simulink model "Bebop2_sim_only_vis"  (R2018a)
settings: Solver=VariableStepAuto  StartTime=0.0  StopTime=20  FixedStep=.05  MaxStep=1  MinStep=0.1  RelTol=50  AbsTol=50
values from neighbouring files (symbols this model uses):
  flightplan = [dist,0,height,deg2rad(090) ... (first row only)    [compare_cubic_spline_1.m]    (also in initialize_race_realtime.m; initialize_race_realtime_backup_cubic.m; plot_sim.m = [ 4.348, -0.278, height, deg2rad(  0); test_b_spline.m)
  FOV = 1.05    [initialize_race_realtime.m]    (also in initialize_race_realtime_backup_cubic.m)
  g = 9.81    [initialize_race_no_realtime.m]    (also in initialize_race_realtime.m; initialize_race_realtime_backup_cubic.m; moving_average_rls_own.m = P(i-1)*meas*(lambda+meas*P(i-1)*meas)^-1)
  gate_size = 1.4    [initialize_race_realtime.m]    (also in initialize_race_realtime_backup_cubic.m)
  gates = sim_gates(:,:,1)    [eval_sim.m]    (also in initialize_race_realtime.m = [dist,0,height,deg2rad(110); initialize_race_realtime_backup_cubic.m = [dist,0,height,deg2rad(110); plot_sim.m)
  init_std_dev = [1.0*ones(1,3),deg2rad(30)]    [initialize_race_realtime.m]    (also in initialize_race_realtime_backup_cubic.m)
  Initial_ori = [0 0 pi/4]    [initialize_race_no_realtime.m]    (also in initialize_race_realtime.m; initialize_race_realtime_backup_cubic.m)
  Initial_pos = [0 0 1]    [Bebop_sim_init.m]    (also in initialize_race_no_realtime.m = [0 -3 2]; initialize_race_realtime.m = [0 -3 2]; initialize_race_realtime_backup_cubic.m = [0 -3 2])
  Initial_vel_e = max_vel*[1,0,0]    [initialize_race_realtime.m]    (also in initialize_race_realtime_backup_cubic.m)
  max_rot_Z = (90)*pi/180    (= 1.57079632679)    [Bebop_sim_init.m]    (also in initialize_race_no_realtime.m = 1.0471975512; initialize_race_realtime.m; initialize_race_realtime_backup_cubic.m; run_batch1.m = list_agility(idx_agility)*max_rot_Z)
  max_theta_X = (40)*pi/180    (= 0.698131700798)    [Bebop_sim_init.m]    (also in initialize_race_no_realtime.m = 0.13962634016; initialize_race_realtime.m = 1.308996939; initialize_race_realtime_backup_cubic.m = 1.308996939; run_batch1.m = list_agility(idx_agility)*max_theta_X)
  max_theta_Y = (40)*pi/180    (= 0.698131700798)    [Bebop_sim_init.m]    (also in initialize_race_no_realtime.m = 0.13962634016; initialize_race_realtime.m = 1.308996939; initialize_race_realtime_backup_cubic.m = 1.308996939; run_batch1.m = list_agility(idx_agility)*max_theta_Y)
  max_v_Z = .5    (= 0.5)    [Bebop_sim_init.m]    (also in initialize_race_no_realtime.m = 1; initialize_race_realtime.m = 3; initialize_race_realtime_backup_cubic.m = 3; run_batch1.m = list_agility(idx_agility)*max_v_Z)
  max_vel = 1.5    [initialize_race_realtime.m]    (also in initialize_race_realtime_backup_cubic.m; run_batch1.m = list_speed(idx_speed); run_batch2.m = list_speed(idx_speed); run_batch3.m = list_speed(idx_speed))
undefined symbols (not defined in the file or in its folder): fspecial, gray, Rec, SDTV
libraries: sharedtransform x9, simulink x4, visiontextngfix x4, visiontransforms x3, vrlib x2, visionanalysis x2, visionconversions x2, aerolibutil x1, visionstatistics x1, visionsinks x1
(part 1 of 2)
settings Model: EnablePacing=on  Creator=vinni  LastModifiedBy=vinni
settings HardwareCC: ProdBitPerLong=64  ProdHWDeviceType=Intel->x86-64 (Linux 64)

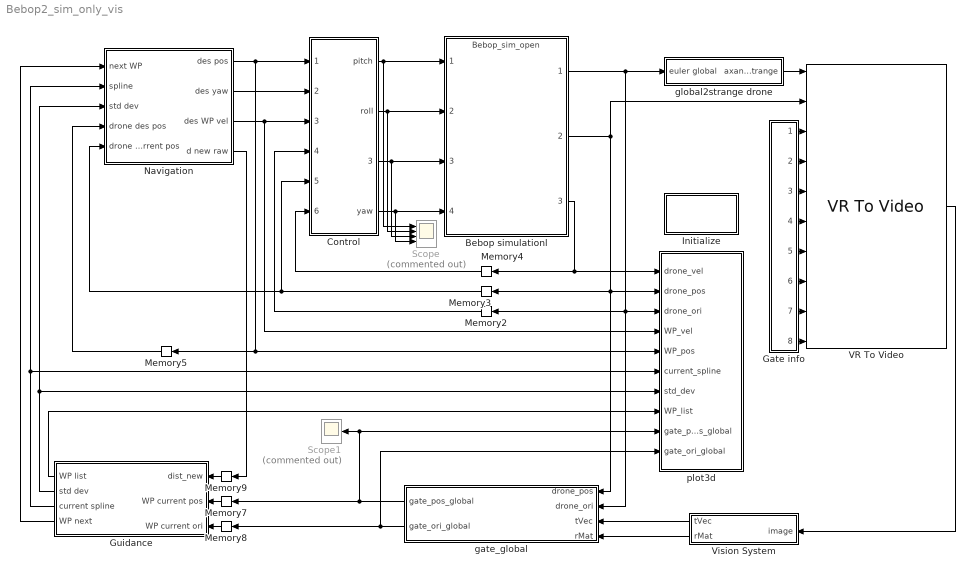
== system Bebop2_sim_only_vis ==
  Bebop simulationl : ModelReference  ModelNameDialog=Bebop_sim_open.slx  SimulationMode=Normal  ModelReferenceVersion=1.35
  Control : Subsystem
  Gate info : Subsystem
  Guidance : Subsystem
  Initialize : Subsystem  TreatAsAtomicUnit=on
  Memory2 : Memory  InitialCondition=Initial_ori
  Memory3 : Memory  InitialCondition=Initial_pos
  Memory4 : Memory  InitialCondition=Initial_vel_e
  Memory5 : Memory
  Memory7 : Memory
  Memory8 : Memory  InitialCondition=zeros(1,3)
  Memory9 : Memory
  Navigation : Subsystem
  Scope : Scope  Commented=on  NumInputPorts=4
  Scope1 : Scope  Commented=on
  VR To Video : vrlib/VR To Video  InstantiateOnLoad=on  SampleTime=0.1000001  ViewEnable=on  RemoteChange=off  RemoteView=off  FieldsWritten=drone.orientation.4.1.1.double#drone.position.3.1.1.double#G1.rotation.4.1.1.double#G1.translation.3.1.1.double#G2.rotation.4.1.1.double#G2.translation.3.1.1.double#G3.rotation.4.1.1.double#G3.translation.3.1.1.double#G4.rotation.4.1.1.double#G4.translation.3.1.1.double  WorldFileName=race_course.wrl  AutoView=off  VideoDimensions=1.5*[200 320]  AllowVariableSize=off  FigureProperties="{'Position', 'Name', 'Viewpoint', 'CameraBound', 'CameraDirection', 'CameraPosition', 'CameraUpVector', 'ZoomFactor', 'Antialiasing', 'Headlight', 'Lighting', 'NavPanel', 'Sound', 'StatusBar', 'Stereo3D', 'Stereo3DCameraOffset', 'Stereo3DHIT', 'ToolBar', 'Textures', 'Transparency', 'Triad', 'Wireframe', 'NavZones', 'NavMode', 'NavSpeed', 'CaptureFileFormat', 'CaptureFileName', 'Record2DCompressMethod', 'Record2DCompressQuality', 'Record2D', 'Record2DFileName', 'Record2DFPS'; [3.0000000000000000e+01   6.0000000000000000e+01   4.8000000000000000e+02   3.0000000000000000e+02], '', '_untitled_1', 'on', [0.0000000000000000e+00   0.0000000000000000e+00  -1.0000000000000000e+00], [0.0000000000000000e+00   0.0000000000000000e+00   0.0000000000000000e+00], [0.0000000000000000e+00   1.0000000000000000e+00   0.0000000000000000e+00], [1.0000000000000000e+00], 'on', 'on', 'on', 'none', 'on', 'off', 'off', [1.0000000149011612e-01], [0.0000000000000000e+00], 'off', 'on', 'on', 'none', 'off', 'off', 'fly', 'normal', 'tif', '%f_anim_%n.tif', 'auto', [7.5000000000000000e+01], 'off', '***video***', 'auto'}"
      settings: SourceProductName=Simulink 3D Animation  SourceProductBaseCode=VR
  Vision System : Subsystem
  gate_global : MATLAB Function  TreatAsAtomicUnit=on
  global2strange drone : Subsystem
  plot3d : MATLAB Function  TreatAsAtomicUnit=on
  wires:
  Bebop simulationl/3 -> plot3d/1(drone_vel), Memory4/1
  Bebop simulationl/2 -> VR To Video/2, Memory3/1, gate_global/1(drone_pos), plot3d/2(drone_pos)
  Bebop simulationl/1 -> global2strange drone/1(euler global), Memory2/1, gate_global/2(drone_ori), plot3d/3(drone_ori)
  gate_global/1(gate_pos_global) -> plot3d/9(gate_pos_global), Scope1/1, Memory7/1
  gate_global/2(gate_ori_global) -> plot3d/10(gate_ori_global), Memory8/1
  VR To Video/1 -> Vision System/1(image)
  Vision System/1(tVec) -> gate_global/3(tVec)
  Vision System/2(rMat) -> gate_global/4(rMat)
  Control/4(yaw) -> Bebop simulationl/4, Scope/4
  Control/3(throttle) -> Bebop simulationl/3, Scope/3
  Control/2(roll) -> Bebop simulationl/2, Scope/2
  Control/1(pitch) -> Bebop simulationl/1, Scope/1
  Memory4/1 -> Control/6(Drone vel)
  Memory2/1 -> Control/4(Drone ori)
  Guidance/3(current spline) -> Navigation/2(spline), plot3d/6(current_spline)
  Memory7/1 -> Guidance/2(WP current pos)
  Memory8/1 -> Guidance/3(WP current ori)
  Memory9/1 -> Guidance/1(dist_new)
  Guidance/1(WP list) -> plot3d/8(WP_list)
  global2strange drone/1(axang strange) -> VR To Video/1
  Gate info/2(P1) -> VR To Video/4
  Gate info/4(P2) -> VR To Video/6
  Gate info/6(P3) -> VR To Video/8
  Gate info/8(P4) -> VR To Video/10
  Gate info/1(O1) -> VR To Video/3
  Gate info/3(O2) -> VR To Video/5
  Gate info/5(O3) -> VR To Video/7
  Gate info/7(O4) -> VR To Video/9
  Memory3/1 -> Control/5(Drone pos), Navigation/5(drone current pos)
  Guidance/2(std dev) -> plot3d/7(std_dev), Navigation/3(std dev)
  Navigation/1(des pos) -> Control/1(WP pos), plot3d/5(WP_pos), Memory5/1
  Navigation/3(des WP vel) -> Control/3(WP vel), plot3d/4(WP_vel)
  Memory5/1 -> Navigation/4(drone des pos)
  Guidance/4(WP next) -> Navigation/1(next WP)
  Navigation/2(des yaw) -> Control/2(des yaw)
  Navigation/4(d new raw) -> Memory9/1

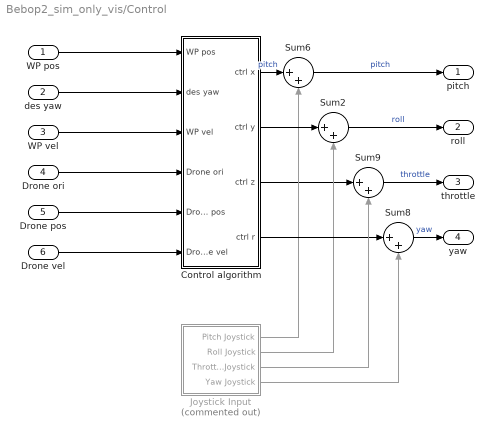
== system Bebop2_sim_only_vis/Control ==
  WP pos : Inport
  des yaw : Inport  Port=2
  WP vel : Inport  Port=3
  Drone ori : Inport  Port=4
  Drone pos : Inport  Port=5
  Drone vel : Inport  Port=6
  Control algorithm : Subsystem
  Joystick Input : Subsystem  Commented=on
  Sum{2,6,8..9} (4 alike) : Sum  Inputs=|++
  pitch : Outport
  roll : Outport  Port=2
  throttle : Outport  Port=3
  yaw : Outport  Port=4
  wires:
  Drone ori/1 -> Control algorithm/4(Drone ori)
  Control algorithm/3(ctrl z) -> Sum9/1
  Joystick Input/2(Roll Joystick) -> Sum2/2
  Joystick Input/4(Yaw Joystick) -> Sum8/2
  Drone pos/1 -> Control algorithm/5(Drone pos)
  Joystick Input/1(Pitch Joystick) -> Sum6/2
  des yaw/1 -> Control algorithm/2(des yaw)
  Sum8/1 -> yaw/1  "yaw"
  Sum6/1 -> pitch/1  "pitch"
  Control algorithm/2(ctrl y) -> Sum2/1
  WP pos/1 -> Control algorithm/1(WP pos)
  Control algorithm/4(ctrl r) -> Sum8/1
  Sum2/1 -> roll/1  "roll"
  WP vel/1 -> Control algorithm/3(WP vel)
  Control algorithm/1(ctrl x) -> Sum6/1  "pitch"
  Drone vel/1 -> Control algorithm/6(Drone vel)
  Sum9/1 -> throttle/1  "throttle"
  Joystick Input/3(Throttle Joystick) -> Sum9/2

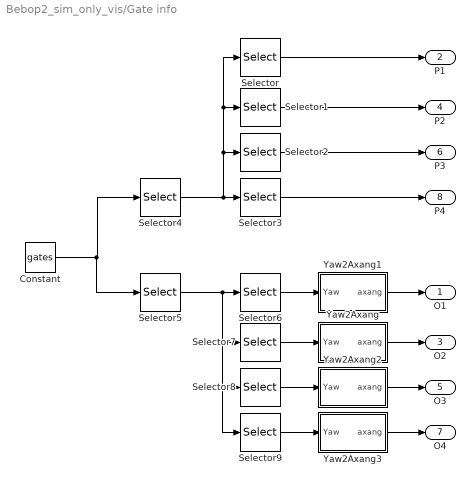
== system Bebop2_sim_only_vis/Gate info ==
  Constant : Constant  Value=gates
  Selector : Selector  NumberOfDimensions=2  InputPortWidth=3  IndexOptions=Index vector (dialog),Select all  Indices=1,1  OutputSizes=1,1
  Selector1 : Selector  NumberOfDimensions=2  InputPortWidth=3  IndexOptions=Index vector (dialog),Select all  Indices=2,1  OutputSizes=1,1
  Selector2 : Selector  NumberOfDimensions=2  InputPortWidth=3  IndexOptions=Index vector (dialog),Select all  Indices=3,1  OutputSizes=1,1
  Selector3 : Selector  NumberOfDimensions=2  InputPortWidth=3  IndexOptions=Index vector (dialog),Select all  Indices=4,1  OutputSizes=1,1
  Selector4 : Selector  NumberOfDimensions=2  InputPortWidth=3  IndexOptions=Select all,Index vector (dialog)  Indices=4,[1 2 3]  OutputSizes=1,1
  Selector5 : Selector  NumberOfDimensions=2  InputPortWidth=3  IndexOptions=Select all,Index vector (dialog)  Indices=4,4  OutputSizes=1,1
  Selector6 : Selector  NumberOfDimensions=2  InputPortWidth=3  IndexOptions=Index vector (dialog),Select all  Indices=1,1  OutputSizes=1,1
  Selector7 : Selector  NumberOfDimensions=2  InputPortWidth=3  IndexOptions=Index vector (dialog),Select all  Indices=2,1  OutputSizes=1,1
  Selector8 : Selector  NumberOfDimensions=2  InputPortWidth=3  IndexOptions=Index vector (dialog),Select all  Indices=3,1  OutputSizes=1,1
  Selector9 : Selector  NumberOfDimensions=2  InputPortWidth=3  IndexOptions=Index vector (dialog),Select all  Indices=4,1  OutputSizes=1,1
  Yaw2Axang : Subsystem
  Yaw2Axang1 : Subsystem
  Yaw2Axang2 : Subsystem
  Yaw2Axang3 : Subsystem
  O1 : Outport
  P1 : Outport  Port=2
  O2 : Outport  Port=3
  P2 : Outport  Port=4
  O3 : Outport  Port=5
  P3 : Outport  Port=6
  O4 : Outport  Port=7
  P4 : Outport  Port=8
  wires:
  Selector/1 -> P1/1
  Selector3/1 -> P4/1
  Selector2/1 -> P3/1
  Selector4/1 -> Selector1/1, Selector/1, Selector2/1, Selector3/1
  Selector1/1 -> P2/1
  Constant/1 -> Selector5/1, Selector4/1
  Selector5/1 -> Selector9/1, Selector8/1, Selector7/1, Selector6/1
  Selector6/1 -> Yaw2Axang1/1(Yaw)
  Selector7/1 -> Yaw2Axang/1(Yaw)
  Selector8/1 -> Yaw2Axang2/1(Yaw)
  Selector9/1 -> Yaw2Axang3/1(Yaw)
  Yaw2Axang1/1(axang) -> O1/1
  Yaw2Axang/1(axang) -> O2/1
  Yaw2Axang2/1(axang) -> O3/1
  Yaw2Axang3/1(axang) -> O4/1

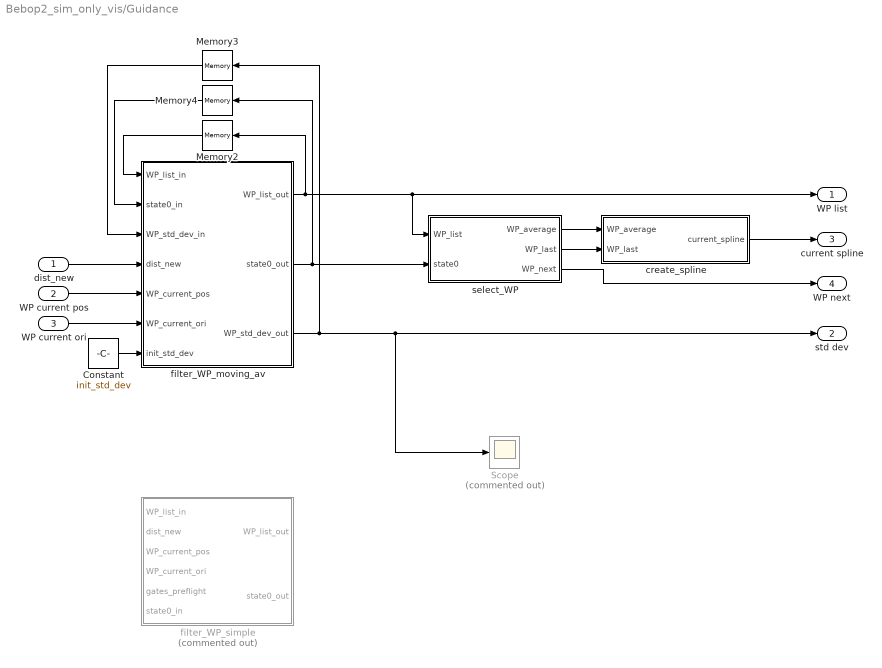
== system Bebop2_sim_only_vis/Guidance ==
  dist_new : Inport
  WP current pos : Inport  Port=2
  WP current ori : Inport  Port=3
  Constant : Constant  Value=init_std_dev
  Memory2 : Memory  InitialCondition=flightplan
  Memory3 : Memory  InitialCondition=init_std_dev
  Memory4 : Memory
  Scope : Scope  Commented=on
  create_spline : MATLAB Function  TreatAsAtomicUnit=on
  filter_WP_moving_av : MATLAB Function  TreatAsAtomicUnit=on
  filter_WP_simple : MATLAB Function  Commented=on  TreatAsAtomicUnit=on
  select_WP : MATLAB Function  TreatAsAtomicUnit=on
  WP list : Outport
  std dev : Outport  Port=2
  current spline : Outport  Port=3
  WP next : Outport  Port=4
  wires:
  WP current ori/1 -> filter_WP_moving_av/6(WP_current_ori)
  create_spline/1(current_spline) -> current spline/1
  select_WP/2(WP_last) -> create_spline/2(WP_last)
  WP current pos/1 -> filter_WP_moving_av/5(WP_current_pos)
  dist_new/1 -> filter_WP_moving_av/4(dist_new)
  select_WP/1(WP_average) -> create_spline/1(WP_average)
  filter_WP_moving_av/1(WP_list_out) -> Memory2/1, WP list/1, select_WP/1(WP_list)
  Memory2/1 -> filter_WP_moving_av/1(WP_list_in)
  filter_WP_moving_av/2(state0_out) -> select_WP/2(state0), Memory4/1
  Memory4/1 -> filter_WP_moving_av/2(state0_in)
  filter_WP_moving_av/3(WP_std_dev_out) -> Scope/1, std dev/1, Memory3/1
  Memory3/1 -> filter_WP_moving_av/3(WP_std_dev_in)
  Constant/1 -> filter_WP_moving_av/7(init_std_dev)
  select_WP/3(WP_next) -> WP next/1

== system Bebop2_sim_only_vis/Initialize ==
  Event Listener : EventListener  DisableCoverage=on  EventName=reset
  reset_plot : MATLAB Function  TreatAsAtomicUnit=on

== system Bebop2_sim_only_vis/Navigation ==
  next WP : Inport
  spline : Inport  Port=2
  std dev : Inport  Port=3
  drone des pos : Inport  Port=4
  drone current pos : Inport  Port=5
  Memory1 : Memory
  calculate desired : Subsystem
  calculate velocity : Subsystem
  set position : Subsystem
  des pos : Outport
  des yaw : Outport  Port=2
  des WP vel : Outport  Port=3
  d new raw : Outport  Port=4
  wires:
  calculate desired/3(WP vel des) -> des WP vel/1
  set position/2(current spline cp) -> calculate desired/3(current spline)
  calculate desired/2(yaw) -> des yaw/1
  calculate velocity/1(dist from gate) -> calculate desired/1(dist from gate)
  drone current pos/1 -> calculate velocity/4(drone current pos), calculate desired/5(drone current pos)
  calculate velocity/2(velocity) -> set position/1(velocity)
  spline/1 -> calculate velocity/1(current spline)
  set position/4(d new raw) -> d new raw/1
  drone des pos/1 -> calculate velocity/2(drone desired pos)
  calculate velocity/3(current spline cp) -> set position/2(current spline)
  set position/3(d new) -> Memory1/1
  calculate desired/1(pos) -> des pos/1
  next WP/1 -> calculate desired/6(WP next)
  set position/1(velocity cp) -> calculate desired/2(vel)
  Memory1/1 -> calculate desired/4(d), set position/3(d old)
  std dev/1 -> calculate velocity/3(std dev)

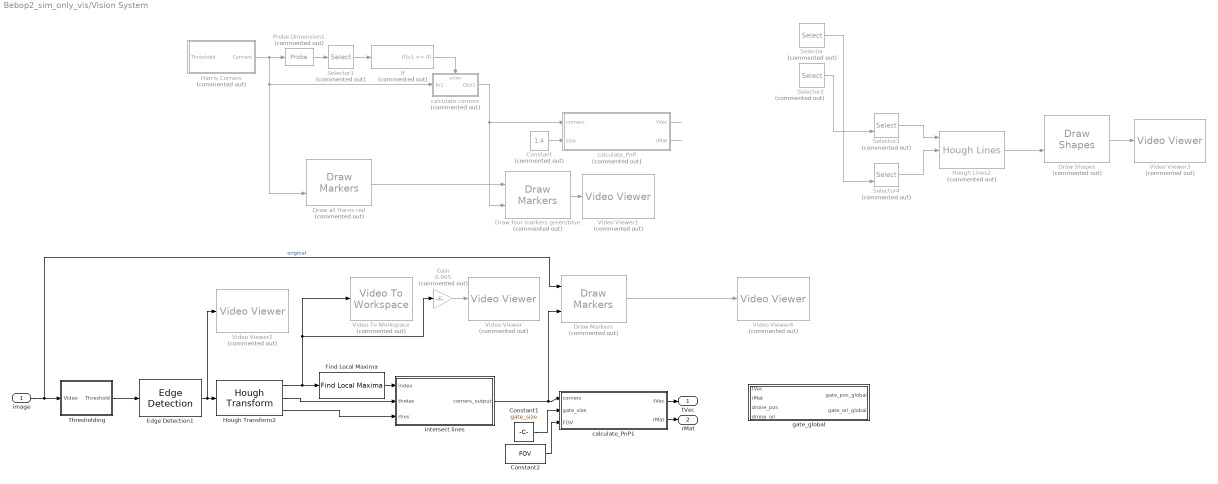
== system Bebop2_sim_only_vis/Vision System ==
  image : Inport
  Constant : Constant  Commented=on  Value=1.4
  Constant1 : Constant  Value=gate_size
  Constant2 : Constant  Value=FOV
  Draw Markers : visiontextngfix/Draw Markers  Commented=on  shape=X-mark  size=10  fill=on  fillClrSource=Specify via dialog  display=User-specified value  intensity=200  color=[255 0 0]  opacity=0.6  viewport=Entire image  antialiasing=off  inType=Obsolete  imagePorts=One multidimensional signal  prodOutputMode=Binary point scaling  prodOutputWordLength=32  prodOutputFracLength=14  memoryMode=Specify word length  memoryWordLength=16  memoryFracLength=14  roundingMode=Floor  overflowMode=off
      settings: SourceProductName=Computer Vision System Toolbox  SourceProductBaseCode=VP
  Draw Shapes : visiontextngfix/Draw Shapes  Commented=on  shape=Lines  fill=off  lineWidth=1  fillClrSource=Specify via dialog  display=White  intensity=200  color=[200 255 100]  opacity=0.6  viewport=Entire image  antialiasing=off  inType=Obsolete  imagePorts=One multidimensional signal  prodOutputMode=Binary point scaling  prodOutputWordLength=32  prodOutputFracLength=14  memoryMode=Specify word length  memoryWordLength=16  memoryFracLength=15  roundingMode=Floor  overflowMode=off
      settings: SourceProductName=Computer Vision System Toolbox
  Draw all Harris red : visiontextngfix/Draw Markers  Commented=on  shape=Circle  size=3  fill=on  fillClrSource=Specify via dialog  display=User-specified value  intensity=200  color=[255 0 0]  opacity=1  viewport=Entire image  antialiasing=off  inType=Obsolete  imagePorts=One multidimensional signal  prodOutputMode=Binary point scaling  prodOutputWordLength=32  prodOutputFracLength=14  memoryMode=Specify word length  memoryWordLength=16  memoryFracLength=14  roundingMode=Floor  overflowMode=off
      settings: SourceProductName=Computer Vision System Toolbox  SourceProductBaseCode=VP
  Draw four markers green/blue : visiontextngfix/Draw Markers  Commented=on  shape=Circle  size=3  fill=on  fillClrSource=Specify via dialog  display=User-specified value  intensity=200  color=[0 255 0; 0 0 255;0 0 255; 0 255 0]  opacity=1  viewport=Entire image  antialiasing=off  inType=Obsolete  imagePorts=One multidimensional signal  prodOutputMode=Binary point scaling  prodOutputWordLength=32  prodOutputFracLength=14  memoryMode=Specify word length  memoryWordLength=16  memoryFracLength=14  roundingMode=Floor  overflowMode=off
      settings: SourceProductName=Computer Vision System Toolbox  SourceProductBaseCode=VP
  Edge Detection1 : visionanalysis/Edge Detection  method=Sobel  outputType=Binary image  userDefinedThreshold=off  thresholdSource=Input port  threshold=20  thresholdTuning=30  edgeThinning=on  threshold_canny=[0.25 0.60]  autoPercent=70  sigma=1  roundingMode=Floor  overflowMode=off  prodOutputMode=Binary point scaling  prodOutputWordLength=32  prodOutputFracLength=8  prodOutputSlope=2^-8  accumSlope=2^-8  outputSlope=2^-4
      settings: SourceProductName=Computer Vision System Toolbox  SourceProductBaseCode=VP
  Find Local Maxima : visionstatistics/Find Local Maxima  num_peaks=8  nhood_size=[7 15]  src_thresh=Obsolete9b  src_thresh_inuse=Specify via dialog  threshold=100  inputIsHough=on  dt_peak=uint32  isOutVarDim=on  dt_count=uint32
      settings: SourceProductName=Computer Vision System Toolbox  SourceProductBaseCode=VP
  Gain : Gain  Commented=on  Gain=0.005
  Harris Corners : Subsystem  Commented=on
  Hough Lines2 : visiontransforms/Hough Lines  Commented=on  sineCompMethod=Trigonometric function  thetaRes=pi/180  firstCoeffMode=Specify word length  firstCoeffWordLength=16  firstCoeffFracLength=15  prodOutputMode=Binary point scaling  prodOutputWordLength=32  prodOutputFracLength=16  roundingMode=Nearest  overflowMode=on
      settings: SourceProductName=Computer Vision System Toolbox  SourceProductBaseCode=VP
  Hough Transform2 : visiontransforms/Hough Transform  theta_res=0.5*pi/180  rho_res=1.5  out_theta_rho=on  outdtmode=double  firstCoeffMode=Binary point scaling  firstCoeffWordLength=16  firstCoeffFracLength=14  secondCoeffMode=Binary point scaling  secondCoeffWordLength=32  secondCoeffFracLength=16  outputMode=Binary point scaling  outputWordLength=16  outputFracLength=0  accumMode=Binary point scaling  accumWordLength=32  accumFracLength=20  prodOutputMode=Binary point scaling  prodOutputWordLength=32  prodOutputFracLength=20  memoryMode=Binary point scaling  memoryWordLength=32  memoryFracLength=16  roundingMode=Nearest  overflowMode=on
      settings: SourceProductName=Computer Vision System Toolbox  SourceProductBaseCode=VP
  If : If  Commented=on  IfExpression=u1 >= 4  ShowElse=off
  Probe Dimension1 : Probe  Commented=on  ProbeWidth=off  ProbeSampleTime=off  ProbeComplexSignal=off  ProbeSignalDimensions=on
  Selector : Selector  Commented=on  NumberOfDimensions=2  InputPortWidth=2  IndexOptions=Select all,Index vector (dialog)  Indices=2,2  OutputSizes=1,1
  Selector1 : Selector  Commented=on  IndexOptions=Index vector (dialog)  Indices=1  OutputSizes=1
  Selector2 : Selector  Commented=on  NumberOfDimensions=2  InputPortWidth=2  IndexOptions=Select all,Index vector (dialog)  Indices=1,1  OutputSizes=1,1
  Selector3 : Selector  Commented=on  NumberOfDimensions=2  InputPortWidth=3  IndexOptions=Select all,Index vector (port)  Indices=[1 3],1  OutputSizes=1,1
  Selector4 : Selector  Commented=on  NumberOfDimensions=2  InputPortWidth=3  IndexOptions=Select all,Index vector (port)  Indices=[1 3],1  OutputSizes=1,1
  Thresholding : Subsystem
  Video To Workspace : visionsinks/Video To Workspace  Commented=on  VariableName=vout  NumInputs=1  DataLimit=10  DecimationFactor=1  LogFi=off  InPortLabels=R|G|B
      settings: SourceProductName=Computer Vision System Toolbox  SourceProductBaseCode=VP
  Video Viewer : VideoViewer  Commented=on  colormapValue=gray(256)  FigPos=[66 898 768 765]
  Video Viewer1 : VideoViewer  Commented=on  colormapValue=gray(256)  FigPos=[823 898 758 735]
  Video Viewer2 : VideoViewer  Commented=on  colormapValue=gray(256)  FigPos=[828 898 768 763]
  Video Viewer3 : VideoViewer  Commented=on  colormapValue=gray(256)  FigPos=[66 898 768 765]
  Video Viewer4 : VideoViewer  Commented=on  colormapValue=gray(256)  FigPos=[808 898 788 735]
  calculate corners : Subsystem  Commented=on  TreatAsAtomicUnit=on
  calculate_PnP : MATLAB Function  Commented=on  TreatAsAtomicUnit=on
  calculate_PnP1 : MATLAB Function  TreatAsAtomicUnit=on
  gate_global : MATLAB Function  TreatAsAtomicUnit=on
  intersect lines : MATLAB Function  TreatAsAtomicUnit=on
  tVec : Outport
  rMat : Outport  Port=2
  wires:
  Probe Dimension1/1 -> Selector1/1
  Draw all Harris red/1 -> Draw four markers green/blue/1
  Harris Corners/1(Corners) -> Probe Dimension1/1, calculate corners/1(In1), Draw all Harris red/2
  Selector1/1 -> If/1
  calculate_PnP/2(rMat) -> ?
  calculate corners/1(Out1) -> Draw four markers green/blue/2, calculate_PnP/1(corners)
  calculate_PnP/1(tVec) -> ?
  Constant/1 -> calculate_PnP/2(size)
  Draw four markers green/blue/1 -> Video Viewer1/1
  If/1 -> calculate corners/Action
  Selector/1 -> Selector4/2
  ? -> Selector2/1, Selector/1  "idx"
  Selector3/1 -> Hough Lines2/1
  Selector4/1 -> Hough Lines2/2
  Hough Transform2/3 -> intersect lines/3(rhos)
  Draw Shapes/1 -> Video Viewer3/1
  Hough Lines2/1 -> Draw Shapes/2
  Hough Transform2/1 -> Find Local Maxima/1, Gain/1, Video To Workspace/1
  Selector2/1 -> Selector3/2
  image/1 -> Draw Markers/1, Thresholding/1("Video ")  "original"
  Thresholding/1(Threshold) -> Edge Detection1/1
  Edge Detection1/1 -> Video Viewer2/1, Hough Transform2/1
  Gain/1 -> Video Viewer/1
  Hough Transform2/2 -> intersect lines/2(thetas)
  Draw Markers/1 -> Video Viewer4/1
  Find Local Maxima/1 -> intersect lines/1(index)
  ? -> Selector3/1  "theta"
  ? -> Selector4/1  "rho"
  ? -> Draw Shapes/1  "original image"
  ? -> Hough Lines2/3  "threshold"
  ? -> Harris Corners/1(Threshold)  "hreshold"
  ? -> Draw all Harris red/1  "original"
  intersect lines/1(corners_output) -> calculate_PnP1/1(corners), Draw Markers/2
  Constant1/1 -> calculate_PnP1/2(gate_size)
  calculate_PnP1/1(tVec) -> tVec/1
  calculate_PnP1/2(rMat) -> rMat/1
  Constant2/1 -> calculate_PnP1/3(FOV)

== system Bebop2_sim_only_vis/global2strange drone ==
  note: rotm2axang(m1*m2)
  note: eul2rotm([-pi/2, 0, pi/2])
  note: eul2rotm([euler(3),euler(2),euler(1)])
  euler global : Inport
  Constant : Constant  Value=pi/2
  Constant1 : Constant  Value=0
  Direction Cosine Matrix to Quaternions : sharedtransform/Direction Cosine Matrix  to Quaternions  aMode=0  action=None  tolerance=eps(2)
      settings: SourceProductName=Aerospace Blockset  SourceProductBaseCode=AE
  Gain : Gain  Gain=-1
  Gain2 : Gain  Gain=-1
  Gain3 : Gain  Gain=[-1,-1,-1,1]
  MATLAB Function : MATLAB Function  Commented=on  TreatAsAtomicUnit=on
  MATLAB Function1 : MATLAB Function  TreatAsAtomicUnit=on
  Matrix Multiply : Product  Multiplication=Matrix(*)
  Rotation Angles to Direction Cosine Matrix : sharedtransform/Rotation Angles to Direction Cosine Matrix  rotationOrder=XYZ  aMode=aMode
      settings: SourceProductBaseCode=AE
  Rotation Angles to Direction Cosine Matrix1 : sharedtransform/Rotation Angles to Direction Cosine Matrix  rotationOrder=XYZ  aMode=aMode
      settings: SourceProductBaseCode=AE
  Vector Concatenate : Concatenate  NumInputs=3
  axang strange : Outport
  wires:
  Constant/1 -> Vector Concatenate/3, Gain/1
  Constant1/1 -> Vector Concatenate/2
  Gain/1 -> Vector Concatenate/1
  Rotation Angles to Direction Cosine Matrix/1 -> Matrix Multiply/2
  euler global/1 -> Gain2/1
  Rotation Angles to Direction Cosine Matrix1/1 -> Matrix Multiply/1
  Matrix Multiply/1 -> Direction Cosine Matrix to Quaternions/1
  MATLAB Function1/1(axang) -> Gain3/1
  Vector Concatenate/1 -> Rotation Angles to Direction Cosine Matrix/1
  Gain2/1 -> Rotation Angles to Direction Cosine Matrix1/1
  Direction Cosine Matrix to Quaternions/1 -> MATLAB Function1/1(q)
  Gain3/1 -> axang strange/1

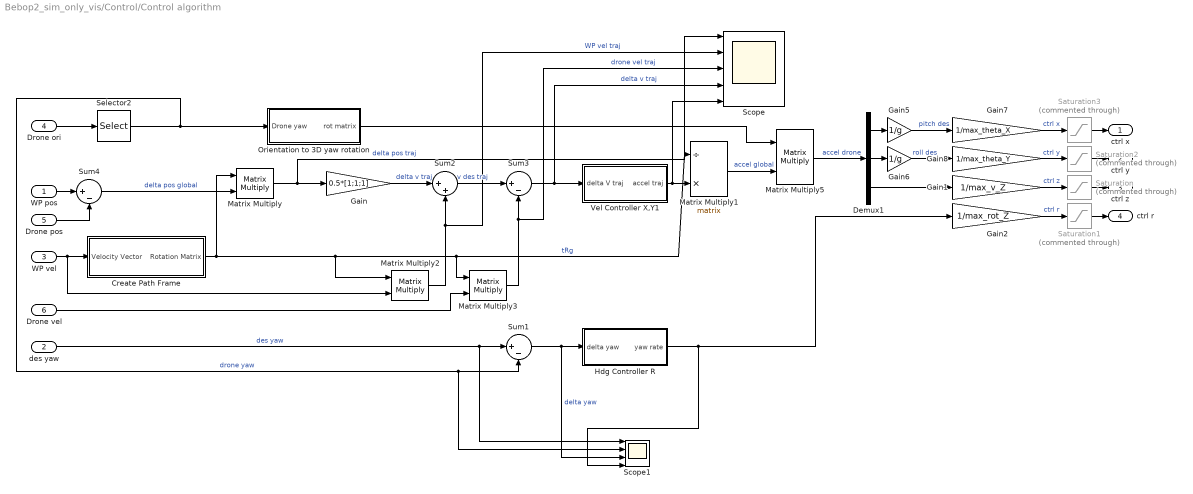
== system Bebop2_sim_only_vis/Control/Control algorithm ==
  WP pos : Inport
  des yaw : Inport  Port=2
  WP vel : Inport  Port=3
  Drone ori : Inport  Port=4
  Drone pos : Inport  Port=5
  Drone vel : Inport  Port=6
  Create Path Frame : Subsystem
  Demux1 : Demux  Outputs=3
  Gain : Gain  Gain=0.5*[1;1;1]
  Gain1 : Gain  Gain=1/max_v_Z
  Gain2 : Gain  Gain=1/max_rot_Z
  Gain5 : Gain  Gain=1/g
  Gain6 : Gain  Gain=1/g
  Gain7 : Gain  Gain=1/max_theta_X
  Gain8 : Gain  Gain=1/max_theta_Y
  Hdg Controller R : Subsystem
  Matrix Multiply{,2..3,5} (4 alike) : Product  Inputs=**  Multiplication=Matrix(*)
  Matrix Multiply1 : Product  Inputs=/*  Multiplication=Matrix(*)
  Orientation to 3D yaw rotation : Subsystem
  Saturation{,1..3} (4 alike) : Saturate  Commented=through  UpperLimit=1  LowerLimit=-1
  Scope : Scope  NumInputPorts=5
  Scope1 : Scope  NumInputPorts=4
  Selector2 : Selector  InputPortWidth=3  IndexOptions=Index vector (dialog)  Indices=3  OutputSizes=1
  Sum1 : Sum  Inputs=|+-
  Sum2 : Sum  Inputs=|++
  Sum3 : Sum  Inputs=|+-
  Sum4 : Sum  Inputs=|+-
  Vel Controller X,Y1 : Subsystem
  ctrl x : Outport
  ctrl y : Outport  Port=2
  ctrl z : Outport  Port=3
  ctrl r : Outport  Port=4
  wires:
  Sum4/1 -> Matrix Multiply/2  "delta pos global"
  Matrix Multiply/1 -> Scope/1, Gain/1  "delta pos traj"
  Create Path Frame/1(Rotation Matrix) -> Matrix Multiply/1, Matrix Multiply2/1, Matrix Multiply1/1, Matrix Multiply3/1  "tRg"
  WP vel/1 -> Matrix Multiply2/2, Create Path Frame/1(Velocity Vector)
  Drone pos/1 -> Sum4/2
  WP pos/1 -> Sum4/1
  Drone vel/1 -> Matrix Multiply3/2
  Gain/1 -> Sum2/1  "delta v traj"
  Drone ori/1 -> Selector2/1
  des yaw/1 -> Scope1/1, Sum1/1  "des yaw"
  Selector2/1 -> Scope1/2, Sum1/2, Orientation to 3D yaw rotation/1(Drone yaw)  "drone yaw"
  Sum1/1 -> Scope1/3, Hdg Controller R/1(delta yaw)  "delta yaw"
  Hdg Controller R/1(yaw rate) -> Scope1/4, Gain2/1
  Sum2/1 -> Sum3/1  "v des traj"
  Matrix Multiply2/1 -> Scope/2, Sum2/2  "WP vel traj"
  Matrix Multiply3/1 -> Scope/3, Sum3/2  "drone vel traj"
  Sum3/1 -> Scope/4, Vel Controller X,Y1/1(delta V traj)  "delta v traj"
  Matrix Multiply1/1 -> Matrix Multiply5/2  "accel global"
  Vel Controller X,Y1/1(accel traj) -> Scope/5, Matrix Multiply1/2
  Orientation to 3D yaw rotation/1(rot matrix) -> Matrix Multiply5/1
  Matrix Multiply5/1 -> Demux1/1  "accel drone"
  Demux1/1 -> Gain5/1
  Demux1/2 -> Gain6/1
  Gain7/1 -> Saturation3/1  "ctrl x"
  Gain8/1 -> Saturation2/1  "ctrl y"
  Saturation2/1 -> ctrl y/1
  Gain5/1 -> Gain7/1  "pitch des"
  Gain6/1 -> Gain8/1  "roll des"
  Saturation3/1 -> ctrl x/1
  Gain1/1 -> Saturation/1  "ctrl z"
  Saturation/1 -> ctrl z/1
  Demux1/3 -> Gain1/1
  Gain2/1 -> Saturation1/1  "ctrl r"
  Saturation1/1 -> ctrl r/1

== system Bebop2_sim_only_vis/Control/Joystick Input ==
  Demux : Demux  Outputs=6
  Gain2 : Gain  Gain=-1
  Joystick Input : vrlib/Joystick Input  joyid=1  adjustports=on  forcefeed=off
      settings: SourceProductBaseCode=VR
  Scope2 : Scope
  Terminator : Terminator
  Terminator1 : Terminator
  Terminator2 : Terminator
  Pitch Joystick : Outport
  Roll Joystick : Outport  Port=2
  Throttle Joystick : Outport  Port=3
  Yaw Joystick : Outport  Port=4
  wires:
  Demux/6 -> Terminator2/1
  Demux/5 -> Terminator1/1
  Demux/2 -> Pitch Joystick/1
  Joystick Input/1 -> Gain2/1
  Demux/1 -> Roll Joystick/1
  Demux/3 -> Yaw Joystick/1
  Gain2/1 -> Scope2/1, Demux/1
  Demux/4 -> Throttle Joystick/1
  Joystick Input/2 -> Terminator/1

== system Bebop2_sim_only_vis/Gate info/Yaw2Axang ==
  Yaw : Inport
  Constant6 : Constant  Value=0
  Constant7 : Constant  Value=-pi/2
  MATLAB Function1 : MATLAB Function  TreatAsAtomicUnit=on
  Rotation Angles to Quaternions : sharedtransform/Rotation Angles to Quaternions  rotationOrder=ZYX  aMode=aMode
      settings: SourceProductName=Aerospace Blockset  SourceProductBaseCode=AE
  Sum : Sum  Inputs=++|
  Vector Concatenate2 : Concatenate  NumInputs=3
  axang : Outport
  wires:
  Sum/1 -> Vector Concatenate2/1
  Constant7/1 -> Sum/1
  Vector Concatenate2/1 -> Rotation Angles to Quaternions/1
  MATLAB Function1/1(axang) -> axang/1
  Rotation Angles to Quaternions/1 -> MATLAB Function1/1(q)
  Constant6/1 -> Vector Concatenate2/2, Vector Concatenate2/3
  Yaw/1 -> Sum/2

== system Bebop2_sim_only_vis/Gate info/Yaw2Axang1 ==
  Yaw : Inport
  Constant6 : Constant  Value=0
  Constant7 : Constant  Value=-pi/2
  MATLAB Function1 : MATLAB Function  TreatAsAtomicUnit=on
  Rotation Angles to Quaternions : sharedtransform/Rotation Angles to Quaternions  rotationOrder=ZYX  aMode=aMode
      settings: SourceProductName=Aerospace Blockset  SourceProductBaseCode=AE
  Sum : Sum  Inputs=++|
  Vector Concatenate2 : Concatenate  NumInputs=3
  axang : Outport
  wires:
  Sum/1 -> Vector Concatenate2/1
  Constant7/1 -> Sum/1
  Vector Concatenate2/1 -> Rotation Angles to Quaternions/1
  MATLAB Function1/1(axang) -> axang/1
  Rotation Angles to Quaternions/1 -> MATLAB Function1/1(q)
  Constant6/1 -> Vector Concatenate2/2, Vector Concatenate2/3
  Yaw/1 -> Sum/2

== system Bebop2_sim_only_vis/Gate info/Yaw2Axang2 ==
  Yaw : Inport
  Constant6 : Constant  Value=0
  Constant7 : Constant  Value=-pi/2
  MATLAB Function1 : MATLAB Function  TreatAsAtomicUnit=on
  Rotation Angles to Quaternions : sharedtransform/Rotation Angles to Quaternions  rotationOrder=ZYX  aMode=aMode
      settings: SourceProductName=Aerospace Blockset  SourceProductBaseCode=AE
  Sum : Sum  Inputs=++|
  Vector Concatenate2 : Concatenate  NumInputs=3
  axang : Outport
  wires:
  Sum/1 -> Vector Concatenate2/1
  Constant7/1 -> Sum/1
  Vector Concatenate2/1 -> Rotation Angles to Quaternions/1
  MATLAB Function1/1(axang) -> axang/1
  Rotation Angles to Quaternions/1 -> MATLAB Function1/1(q)
  Constant6/1 -> Vector Concatenate2/2, Vector Concatenate2/3
  Yaw/1 -> Sum/2

== system Bebop2_sim_only_vis/Gate info/Yaw2Axang3 ==
  Yaw : Inport
  Constant6 : Constant  Value=0
  Constant7 : Constant  Value=-pi/2
  MATLAB Function1 : MATLAB Function  TreatAsAtomicUnit=on
  Rotation Angles to Quaternions : sharedtransform/Rotation Angles to Quaternions  rotationOrder=ZYX  aMode=aMode
      settings: SourceProductName=Aerospace Blockset  SourceProductBaseCode=AE
  Sum : Sum  Inputs=++|
  Vector Concatenate2 : Concatenate  NumInputs=3
  axang : Outport
  wires:
  Sum/1 -> Vector Concatenate2/1
  Constant7/1 -> Sum/1
  Vector Concatenate2/1 -> Rotation Angles to Quaternions/1
  MATLAB Function1/1(axang) -> axang/1
  Rotation Angles to Quaternions/1 -> MATLAB Function1/1(q)
  Constant6/1 -> Vector Concatenate2/2, Vector Concatenate2/3
  Yaw/1 -> Sum/2

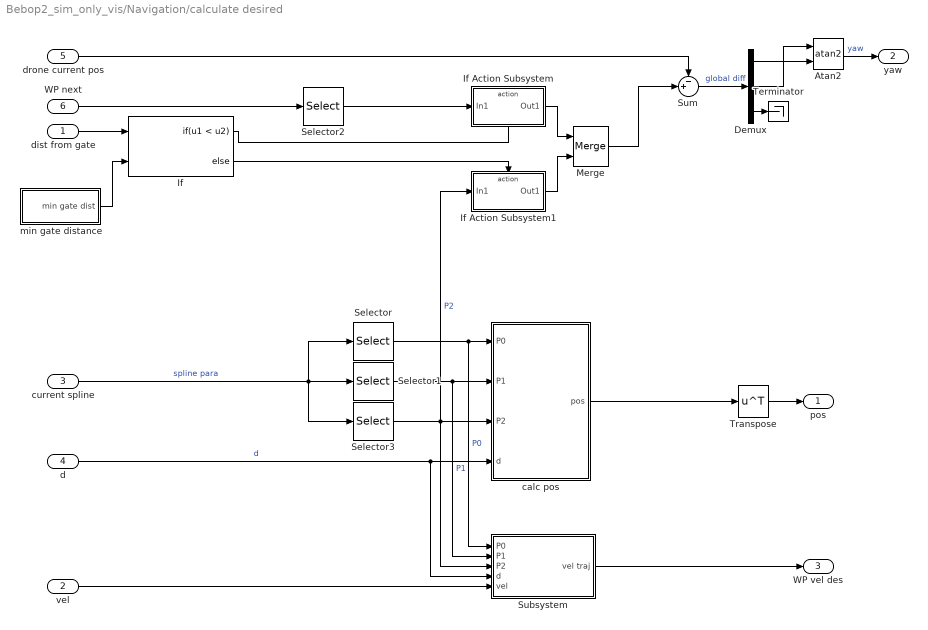
== system Bebop2_sim_only_vis/Navigation/calculate desired ==
  dist from gate : Inport
  vel : Inport  Port=2
  current spline : Inport  Port=3
  d : Inport  Port=4
  drone current pos : Inport  Port=5
  WP next : Inport  Port=6
  Atan2 : Trigonometry  Operator=atan2
  Demux : Demux  Outputs=3
  If : If  NumInputs=2  IfExpression=u1 < u2
  If Action Subsystem : Subsystem  TreatAsAtomicUnit=on
  If Action Subsystem1 : Subsystem  TreatAsAtomicUnit=on
  Merge : Merge
  Selector : Selector  NumberOfDimensions=2  InputPortWidth=3  IndexOptions=Index vector (dialog),Index vector (dialog)  Indices=1,[1 2 3]  OutputSizes=1,1
  Selector1 : Selector  NumberOfDimensions=2  InputPortWidth=3  IndexOptions=Index vector (dialog),Index vector (dialog)  Indices=2,[1 2 3]  OutputSizes=1,1
  Selector2 : Selector  NumberOfDimensions=2  InputPortWidth=4  IndexOptions=Select all,Index vector (dialog)  Indices=[1 2 3],[1 2 3]  OutputSizes=1,1
  Selector3 : Selector  NumberOfDimensions=2  InputPortWidth=3  IndexOptions=Index vector (dialog),Index vector (dialog)  Indices=3,[1 2 3]  OutputSizes=1,1
  Subsystem : Subsystem
  Sum : Sum  Inputs=-+|
  Terminator : Terminator
  Transpose : Math  Operator=transpose  SaturateOnIntegerOverflow=on
  calc pos : Subsystem
  min gate distance : Subsystem
  pos : Outport
  yaw : Outport  Port=2
  WP vel des : Outport  Port=3
  wires:
  current spline/1 -> Selector3/1, Selector1/1, Selector/1  "spline para"
  Selector/1 -> Subsystem/1(P0), calc pos/1(P0)  "P0"
  Selector1/1 -> Subsystem/2(P1), calc pos/2(P1)  "P1"
  Selector3/1 -> If Action Subsystem1/1(In1), Subsystem/3(P2), calc pos/3(P2)  "P2"
  d/1 -> calc pos/4(d), Subsystem/4(d)  "d"
  calc pos/1(pos) -> Transpose/1
  Sum/1 -> Demux/1  "global diff"
  Demux/2 -> Atan2/1
  Demux/1 -> Atan2/2
  Demux/3 -> Terminator/1
  Atan2/1 -> yaw/1  "yaw"
  vel/1 -> Subsystem/5(vel)
  Subsystem/1(vel traj) -> WP vel des/1
  Transpose/1 -> pos/1
  drone current pos/1 -> Sum/1
  dist from gate/1 -> If/1
  min gate distance/1(min gate dist) -> If/2
  If/1 -> If Action Subsystem/Action
  If/2 -> If Action Subsystem1/Action
  WP next/1 -> Selector2/1
  If Action Subsystem/1(Out1) -> Merge/1
  If Action Subsystem1/1(Out1) -> Merge/2
  Merge/1 -> Sum/2
  Selector2/1 -> If Action Subsystem/1(In1)

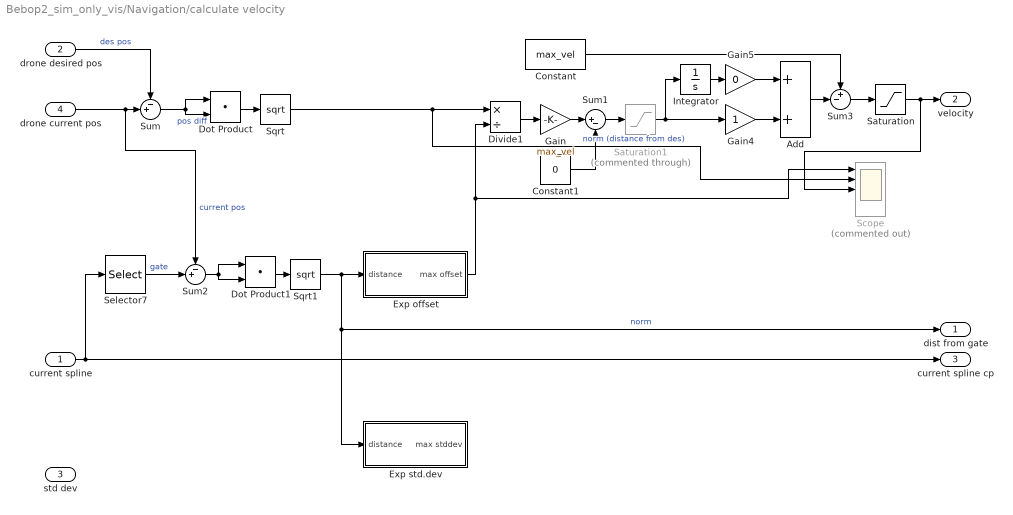
== system Bebop2_sim_only_vis/Navigation/calculate velocity ==
  current spline : Inport
  drone desired pos : Inport  Port=2
  std dev : Inport  Port=3
  drone current pos : Inport  Port=4
  Add : Sum
  Constant : Constant  Value=max_vel
  Constant1 : Constant  Value=0
  Divide1 : Product  Inputs=*/
  Dot Product : DotProduct  InputSameDT=on  OutDataTypeStr=Inherit: Inherit via internal rule
  Dot Product1 : DotProduct  InputSameDT=on  OutDataTypeStr=Inherit: Inherit via internal rule
  Exp offset : Subsystem
  Exp std.dev : Subsystem
  Gain : Gain  Gain=max_vel
  Gain4 : Gain
  Gain5 : Gain  Gain=0
  Integrator : Integrator
  Saturation : Saturate  UpperLimit=max_vel  LowerLimit=0.01
  Saturation1 : Saturate  Commented=through  UpperLimit=1  LowerLimit=0
  Scope : Scope  Commented=on  NumInputPorts=5
  Selector7 : Selector  NumberOfDimensions=2  InputPortWidth=3  IndexOptions=Index vector (dialog),Index vector (dialog)  Indices=3,[1 2 3]  OutputSizes=1,1
  Sqrt : Sqrt  SaturateOnIntegerOverflow=on
  Sqrt1 : Sqrt  SaturateOnIntegerOverflow=on
  Sum : Sum  Inputs=-+|
  Sum1 : Sum  Inputs=|+-
  Sum2 : Sum  Inputs=-+|
  Sum3 : Sum  Inputs=+-|
  dist from gate : Outport
  velocity : Outport  Port=2
  current spline cp : Outport  Port=3
  wires:
  drone current pos/1 -> Sum2/1, Sum/2  "current pos"
  drone desired pos/1 -> Sum/1  "des pos"
  Dot Product/1 -> Sqrt/1
  Sum/1 -> Dot Product/2, Dot Product/1  "pos diff"
  Sqrt/1 -> Scope/2, Divide1/1  "norm (distance from des)"
  current spline/1 -> current spline cp/1, Selector7/1
  Selector7/1 -> Sum2/2  "gate"
  Sqrt1/1 -> Exp std.dev/1(distance), dist from gate/1, Exp offset/1(distance)  "norm"
  Sum2/1 -> Dot Product1/1, Dot Product1/2
  Dot Product1/1 -> Sqrt1/1
  Exp offset/1(max offset) -> Divide1/2, Scope/1
  Divide1/1 -> Gain/1
  Gain/1 -> Sum1/1
  Constant1/1 -> Sum1/2
  Sum1/1 -> Saturation1/1
  Constant/1 -> Sum3/1
  Sum3/1 -> Saturation/1
  Saturation/1 -> Scope/3, velocity/1
  Gain4/1 -> Add/2
  Saturation1/1 -> Integrator/1, Gain4/1
  Integrator/1 -> Gain5/1
  Gain5/1 -> Add/1
  Add/1 -> Sum3/2

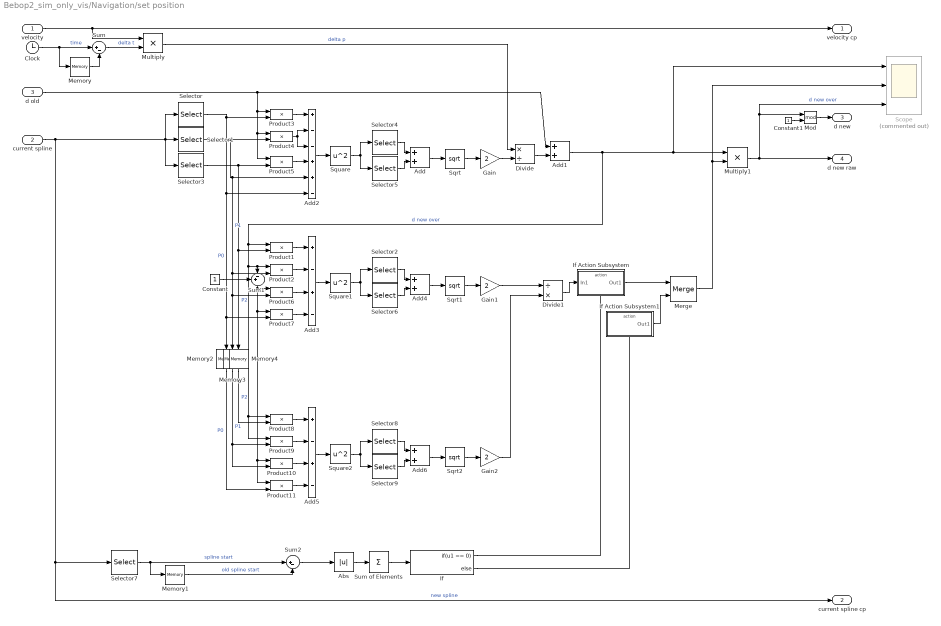
== system Bebop2_sim_only_vis/Navigation/set position ==
  velocity : Inport
  current spline : Inport  Port=2
  d old : Inport  Port=3
  Abs : Abs
  Add{,1,4,6} (4 alike) : Sum
  Add2 : Sum  Inputs=+--++-
  Add3 : Sum  Inputs=+-+-
  Add5 : Sum  Inputs=+-+-
  Clock : Clock
  Constant : Constant
  Constant1 : Constant
  Divide : Product  Inputs=*/
  Divide1 : Product  Inputs=/*
  Gain : Gain  Gain=2
  Gain1 : Gain  Gain=2
  Gain2 : Gain  Gain=2
  If : If  IfExpression=u1 == 0
  If Action Subsystem : Subsystem  TreatAsAtomicUnit=on
  If Action Subsystem1 : Subsystem  TreatAsAtomicUnit=on
  Memory{,1..4} (5 alike) : Memory
  Merge : Merge
  Mod : Math  Operator=mod  SaturateOnIntegerOverflow=on
  Multiply : Product
  Multiply1 : Product
  Product{1..11} (11 alike) : Product
  Scope : Scope  Commented=on  NumInputPorts=3
  Selector : Selector  NumberOfDimensions=2  InputPortWidth=3  IndexOptions=Index vector (dialog),Index vector (dialog)  Indices=1,[1 2 3]  OutputSizes=1,1
  Selector1 : Selector  NumberOfDimensions=2  InputPortWidth=3  IndexOptions=Index vector (dialog),Index vector (dialog)  Indices=2,[1 2 3]  OutputSizes=1,1
  Selector2 : Selector  InputPortWidth=3  IndexOptions=Index vector (dialog)  Indices=2  OutputSizes=1
  Selector3 : Selector  NumberOfDimensions=2  InputPortWidth=3  IndexOptions=Index vector (dialog),Index vector (dialog)  Indices=3,[1 2 3]  OutputSizes=1,1
  Selector4 : Selector  InputPortWidth=3  IndexOptions=Index vector (dialog)  Indices=2  OutputSizes=1
  Selector5 : Selector  InputPortWidth=3  IndexOptions=Index vector (dialog)  Indices=1  OutputSizes=1
  Selector6 : Selector  InputPortWidth=3  IndexOptions=Index vector (dialog)  Indices=1  OutputSizes=1
  Selector7 : Selector  NumberOfDimensions=2  InputPortWidth=3  IndexOptions=Index vector (dialog),Index vector (dialog)  Indices=1,[1 2 3]  OutputSizes=1,1
  Selector8 : Selector  InputPortWidth=3  IndexOptions=Index vector (dialog)  Indices=2  OutputSizes=1
  Selector9 : Selector  InputPortWidth=3  IndexOptions=Index vector (dialog)  Indices=1  OutputSizes=1
  Sqrt : Sqrt  SaturateOnIntegerOverflow=on
  Sqrt1 : Sqrt  SaturateOnIntegerOverflow=on
  Sqrt2 : Sqrt  SaturateOnIntegerOverflow=on
  Square : Math  Operator=square  SaturateOnIntegerOverflow=on
  Square1 : Math  Operator=square  SaturateOnIntegerOverflow=on
  Square2 : Math  Operator=square  SaturateOnIntegerOverflow=on
  Sum : Sum  Inputs=|+-
  Sum of Elements : Sum  Inputs=+
  Sum1 : Sum  Inputs=+-|
  Sum2 : Sum  Inputs=|+-
  velocity cp : Outport
  current spline cp : Outport  Port=2
  d new : Outport  Port=3
  d new raw : Outport  Port=4
  wires:
  Clock/1 -> Sum/1, Memory/1  "time"
  Memory/1 -> Sum/2
  Sum/1 -> Multiply/2  "delta t"
  velocity/1 -> velocity cp/1, Multiply/1
  Multiply/1 -> Divide/1  "delta p"
  Selector1/1 -> Product4/2, Add2/5, Product2/2, Memory3/1, Product6/2  "P1"
  Selector/1 -> Product3/2, Add2/6, Memory2/1, Product7/2  "P0"
  current spline/1 -> current spline cp/1, Selector7/1, Selector/1, Selector3/1, Selector1/1  "new spline"
  Selector5/1 -> Add/2
  d old/1 -> Add1/1, Product3/1, Product4/1, Product5/1
  Add2/1 -> Square/1
  Selector4/1 -> Add/1
  Selector3/1 -> Product5/2, Memory4/1, Product1/2  "P2"
  Product4/1 -> Add2/2, Add2/3
  Product3/1 -> Add2/1
  Product5/1 -> Add2/4
  Square/1 -> Selector5/1, Selector4/1
  Add/1 -> Sqrt/1
  Sqrt/1 -> Gain/1
  Gain/1 -> Divide/2
  Divide/1 -> Add1/2
  Multiply1/1 -> Scope/3, Mod/1, d new raw/1  "d new over"
  Memory1/1 -> Sum2/2  "old spline start"
  Product1/1 -> Add3/1
  Product2/1 -> Add3/2
  Product6/1 -> Add3/3
  Product7/1 -> Add3/4
  Constant/1 -> Sum1/1
  Selector6/1 -> Add4/2
  Square1/1 -> Selector6/1, Selector2/1
  Sqrt1/1 -> Gain1/1
  Selector2/1 -> Add4/1
  Gain1/1 -> Divide1/1
  Add4/1 -> Sqrt1/1
  Add3/1 -> Square1/1
  If/1 -> If Action Subsystem/Action
  Divide1/1 -> If Action Subsystem/1(In1)
  If Action Subsystem1/1(Out1) -> Merge/2
  Selector7/1 -> Sum2/1, Memory1/1  "spline start"
  Sum2/1 -> Abs/1
  Sum of Elements/1 -> If/1
  Abs/1 -> Sum of Elements/1
  If/2 -> If Action Subsystem1/Action
  If Action Subsystem/1(Out1) -> Merge/1
  Merge/1 -> Scope/2, Multiply1/2
  Memory2/1 -> Product11/2  "P0"
  Selector8/1 -> Add6/1
  Gain2/1 -> Divide1/2
  Product9/1 -> Add5/2
  Add6/1 -> Sqrt2/1
  Memory4/1 -> Product8/2  "P2"
  Sqrt2/1 -> Gain2/1
  Add1/1 -> Product1/1, Product8/1, Product9/1, Product2/1, Sum1/2, Scope/1, Multiply1/1  "d new over"
  Sum1/1 -> Product11/1, Product10/1, Product7/1, Product6/1
  Product8/1 -> Add5/1
  Product10/1 -> Add5/3
  Selector9/1 -> Add6/2
  Product11/1 -> Add5/4
  Add5/1 -> Square2/1
  Square2/1 -> Selector9/1, Selector8/1
  Memory3/1 -> Product9/2, Product10/2  "P1"
  Mod/1 -> d new/1
  Constant1/1 -> Mod/2

== system Bebop2_sim_only_vis/Vision System/Harris Corners ==
  Threshold : Inport
  Corner Detection : visionanalysis/Corner Detection  method=Harris corner detection (Harris & Stephens)  factor=0.01  filter=fspecial('gaussian', [1 9], 3)  thrInten=0.1  thrAngle=157.5  output=Obsolete9b  outputInUse=Corner location  maxNum=5  thrMetric=0.01  neighborSize=[25 25]  isOutVarDim=on  accumMode=Binary point scaling  accumWordLength=32  accumFracLength=0  prodOutputMode=Binary point scaling  prodOutputWordLength=32  prodOutputFracLength=0  memoryMode=Binary point scaling  memoryWordLength=32  memoryFracLength=0  firstCoeffMode=Specify word length  firstCoeffWordLength=16  firstCoeffFracLength=17  roundingMode=Floor  overflowMode=off
      settings: SourceProductName=Computer Vision System Toolbox  SourceProductBaseCode=VP
  Gaussian Pyramid : visiontransforms/Gaussian Pyramid  Commented=on  operation=Expand  level=1  source=Specify via dialog  a=0.375  coef=fspecial('gaussian', [1 9], 3)  hiddenCoef=fspecial('gaussian', [1 9], 3)  firstCoeffMode=Specify word length  firstCoeffWordLength=16  firstCoeffFracLength=17  outputMode=Binary point scaling  outputWordLength=32  outputFracLength=10  prodOutputMode=Binary point scaling  prodOutputWordLength=32  prodOutputFracLength=10  roundingMode=Floor  overflowMode=off
      settings: SourceProductName=Computer Vision System Toolbox  SourceProductBaseCode=VP
  Video Viewer2 : VideoViewer  Commented=on  colormapValue=gray(256)  FigPos=[76 898 768 763]
  Corners : Outport
  wires:
  Threshold/1 -> Gaussian Pyramid/1, Corner Detection/1
  Gaussian Pyramid/1 -> Video Viewer2/1
  Corner Detection/1 -> Corners/1

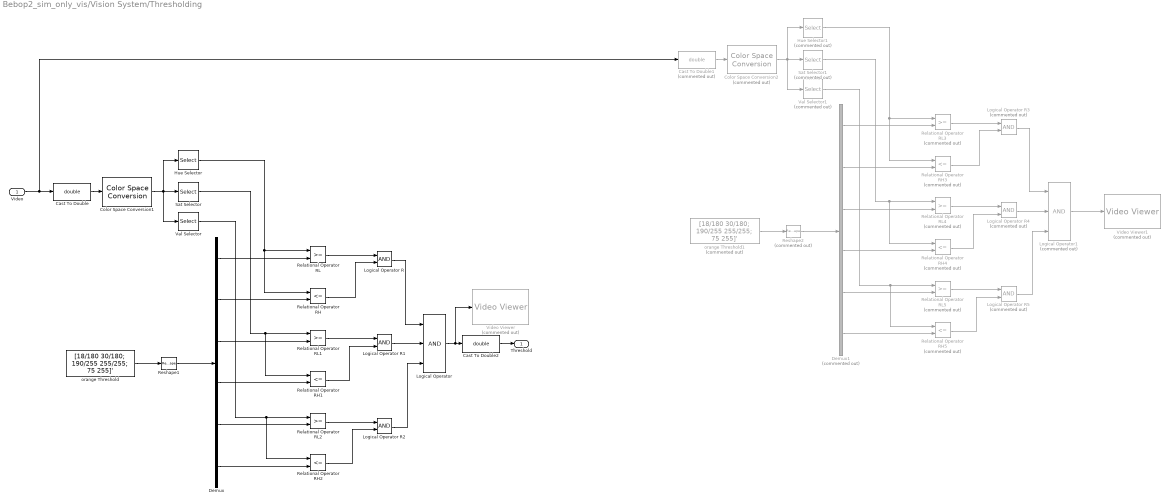
== system Bebop2_sim_only_vis/Vision System/Thresholding ==
  "Video " : Inport
  Cast To Double : DataTypeConversion  OutDataTypeStr=double
  Cast To Double1 : DataTypeConversion  Commented=on  OutDataTypeStr=double
  Cast To Double2 : DataTypeConversion  OutDataTypeStr=double
  Color Space Conversion1 : visionconversions/Color Space  Conversion  conversion=Obsolete  conversionActive=R'G'B' to HSV  wp_str=D65  rec=Rec. 601 (SDTV)  sys=1125/60/2:1  imagePorts=One multidimensional signal
      settings: SourceProductName=Computer Vision System Toolbox
  Color Space Conversion2 : visionconversions/Color Space  Conversion  Commented=on  conversion=Obsolete  conversionActive=R'G'B' to HSV  wp_str=D65  rec=Rec. 601 (SDTV)  sys=1125/60/2:1  imagePorts=One multidimensional signal
      settings: SourceProductName=Computer Vision System Toolbox
  Demux : Demux  Outputs=6
  Demux1 : Demux  Commented=on  Outputs=6
  Hue Selector : Selector  NumberOfDimensions=3  InputPortWidth=3  IndexOptions=Select all,Select all,Index vector (dialog)  Indices=[1 3],1,1  OutputSizes=1,1,1
  Hue Selector1 : Selector  Commented=on  NumberOfDimensions=3  InputPortWidth=3  IndexOptions=Select all,Select all,Index vector (dialog)  Indices=[1 3],1,1  OutputSizes=1,1,1
  Logical Operator : Logic  Inputs=3  AllPortsSameDT=off  OutDataTypeStr=boolean
  Logical Operator R : Logic  AllPortsSameDT=off  OutDataTypeStr=boolean
  Logical Operator R1 : Logic  AllPortsSameDT=off  OutDataTypeStr=boolean
  Logical Operator R2 : Logic  AllPortsSameDT=off  OutDataTypeStr=boolean
  Logical Operator R3 : Logic  Commented=on  AllPortsSameDT=off  OutDataTypeStr=boolean
  Logical Operator R4 : Logic  Commented=on  AllPortsSameDT=off  OutDataTypeStr=boolean
  Logical Operator R5 : Logic  Commented=on  AllPortsSameDT=off  OutDataTypeStr=boolean
  Logical Operator1 : Logic  Commented=on  Inputs=3  AllPortsSameDT=off  OutDataTypeStr=boolean
  Relational Operator RH : RelationalOperator  Operator=<=  OutDataTypeStr=boolean  RndMeth=Nearest
  Relational Operator RH1 : RelationalOperator  Operator=<=  OutDataTypeStr=boolean  RndMeth=Nearest
  Relational Operator RH2 : RelationalOperator  Operator=<=  OutDataTypeStr=boolean  RndMeth=Nearest
  Relational Operator RH3 : RelationalOperator  Commented=on  Operator=<=  OutDataTypeStr=boolean  RndMeth=Nearest
  Relational Operator RH4 : RelationalOperator  Commented=on  Operator=<=  OutDataTypeStr=boolean  RndMeth=Nearest
  Relational Operator RH5 : RelationalOperator  Commented=on  Operator=<=  OutDataTypeStr=boolean  RndMeth=Nearest
  Relational Operator RL : RelationalOperator  OutDataTypeStr=boolean  RndMeth=Nearest
  Relational Operator RL1 : RelationalOperator  OutDataTypeStr=boolean  RndMeth=Nearest
  Relational Operator RL2 : RelationalOperator  OutDataTypeStr=boolean  RndMeth=Nearest
  Relational Operator RL3 : RelationalOperator  Commented=on  OutDataTypeStr=boolean  RndMeth=Nearest
  Relational Operator RL4 : RelationalOperator  Commented=on  OutDataTypeStr=boolean  RndMeth=Nearest
  Relational Operator RL5 : RelationalOperator  Commented=on  OutDataTypeStr=boolean  RndMeth=Nearest
  Reshape1 : Reshape
  Reshape2 : Reshape  Commented=on
  Sat Selector : Selector  NumberOfDimensions=3  InputPortWidth=3  IndexOptions=Select all,Select all,Index vector (dialog)  Indices=[1 3],1,2  OutputSizes=1,1,1
  Sat Selector1 : Selector  Commented=on  NumberOfDimensions=3  InputPortWidth=3  IndexOptions=Select all,Select all,Index vector (dialog)  Indices=[1 3],1,2  OutputSizes=1,1,1
  Val Selector : Selector  NumberOfDimensions=3  InputPortWidth=3  IndexOptions=Select all,Select all,Index vector (dialog)  Indices=[1 3],1,3  OutputSizes=1,1,1
  Val Selector1 : Selector  Commented=on  NumberOfDimensions=3  InputPortWidth=3  IndexOptions=Select all,Select all,Index vector (dialog)  Indices=[1 3],1,3  OutputSizes=1,1,1
  Video Viewer : VideoViewer  Commented=on  colormapValue=gray(256)  FigPos=[833 898 768 793]
  Video Viewer1 : VideoViewer  Commented=on  colormapValue=gray(256)  FigPos=[823 898 778 793]
  orange Threshold : Constant  Value=[18/180 30/180; 190/255 255/255; 75 255]'  OutDataTypeStr=double
  orange Threshold1 : Constant  Commented=on  Value=[18/180 30/180; 190/255 255/255; 75 255]'  OutDataTypeStr=double
  Threshold : Outport
  wires:
  Color Space Conversion1/1 -> Val Selector/1, Sat Selector/1, Hue Selector/1
  Demux/6 -> Relational Operator RH2/2
  Val Selector/1 -> Relational Operator RH2/1, Relational Operator RL2/1
  Demux/3 -> Relational Operator RL1/2
  Relational Operator RL/1 -> Logical Operator R/1
  Demux/2 -> Relational Operator RH/2
  orange Threshold/1 -> Reshape1/1
  Cast To Double/1 -> Color Space Conversion1/1
  Demux/5 -> Relational Operator RL2/2
  Hue Selector/1 -> Relational Operator RH/1, Relational Operator RL/1
  Logical Operator R/1 -> Logical Operator/1
  Relational Operator RH/1 -> Logical Operator R/2
  Demux/1 -> Relational Operator RL/2
  Demux/4 -> Relational Operator RH1/2
  Reshape1/1 -> Demux/1
  Logical Operator R1/1 -> Logical Operator/2
  Relational Operator RH1/1 -> Logical Operator R1/2
  Sat Selector/1 -> Relational Operator RH1/1, Relational Operator RL1/1
  Relational Operator RL1/1 -> Logical Operator R1/1
  Relational Operator RH2/1 -> Logical Operator R2/2
  Relational Operator RL2/1 -> Logical Operator R2/1
  Logical Operator R2/1 -> Logical Operator/3
  Logical Operator/1 -> Video Viewer/1, Cast To Double2/1
  Demux1/5 -> Relational Operator RL5/2
  Relational Operator RH3/1 -> Logical Operator R3/2
  orange Threshold1/1 -> Reshape2/1
  Demux1/1 -> Relational Operator RL3/2
  Relational Operator RH4/1 -> Logical Operator R4/2
  Demux1/4 -> Relational Operator RH4/2
  Relational Operator RH5/1 -> Logical Operator R5/2
  Logical Operator R5/1 -> Logical Operator1/3
  Relational Operator RL4/1 -> Logical Operator R4/1
  Demux1/6 -> Relational Operator RH5/2
  Demux1/2 -> Relational Operator RH3/2
  Reshape2/1 -> Demux1/1
  Logical Operator1/1 -> Video Viewer1/1
  Hue Selector1/1 -> Relational Operator RH3/1, Relational Operator RL3/1
  Color Space Conversion2/1 -> Val Selector1/1, Sat Selector1/1, Hue Selector1/1
  Logical Operator R3/1 -> Logical Operator1/1
  Cast To Double1/1 -> Color Space Conversion2/1
  Demux1/3 -> Relational Operator RL4/2
  Relational Operator RL3/1 -> Logical Operator R3/1
  Val Selector1/1 -> Relational Operator RH5/1, Relational Operator RL5/1
  Relational Operator RL5/1 -> Logical Operator R5/1
  Logical Operator R4/1 -> Logical Operator1/2
  "Video "/1 -> Cast To Double1/1, Cast To Double/1
  Sat Selector1/1 -> Relational Operator RH4/1, Relational Operator RL4/1
  Cast To Double2/1 -> Threshold/1

== system Bebop2_sim_only_vis/Vision System/calculate corners ==
  In1 : Inport
  Action Port : ActionPort  PropagateVarSize=During execution  ActionType=then
  calculate corners : MATLAB Function  TreatAsAtomicUnit=on
  Out1 : Outport
  wires:
  In1/1 -> calculate corners/1(corners)
  calculate corners/1(corners_four) -> Out1/1

== system Bebop2_sim_only_vis/Control/Control algorithm/Create Path Frame ==
  Velocity Vector : Inport
  Invert 3x3 Matrix : aerolibutil/Invert  3x3 Matrix
  Make X Vector : Subsystem
  Make Y Vector : Subsystem
  Make Z Vector : Subsystem
  Matrix Concatenate : Concatenate  NumInputs=3  Mode=Multidimensional array  ConcatenateDimension=2
  Rotation Matrix : Outport
  wires:
  Velocity Vector/1 -> Make Z Vector/1(Velocity Vector), Make X Vector/1(Velocity Vector), Make Y Vector/1(Velocity Vector)
  Make Y Vector/1(Y Vector) -> Matrix Concatenate/2
  Make X Vector/1(X Vector) -> Matrix Concatenate/1
  Make Z Vector/1(Z Vector) -> Matrix Concatenate/3
  Matrix Concatenate/1 -> Invert 3x3 Matrix/1
  Invert 3x3 Matrix/1 -> Rotation Matrix/1
